simulink model "MPM"  (R2018b)
settings: Solver=VariableStepAuto  StartTime=0.0  StopTime=10.0  RelTol=1e-3
undefined symbols (not defined in the file): Cw, Cwc, Jt, Jw, k1, k2, k3, k4, Mt, R3, R4, Rg, Rw
settings Model: Creator=HYJ  LastModifiedBy=HYJ

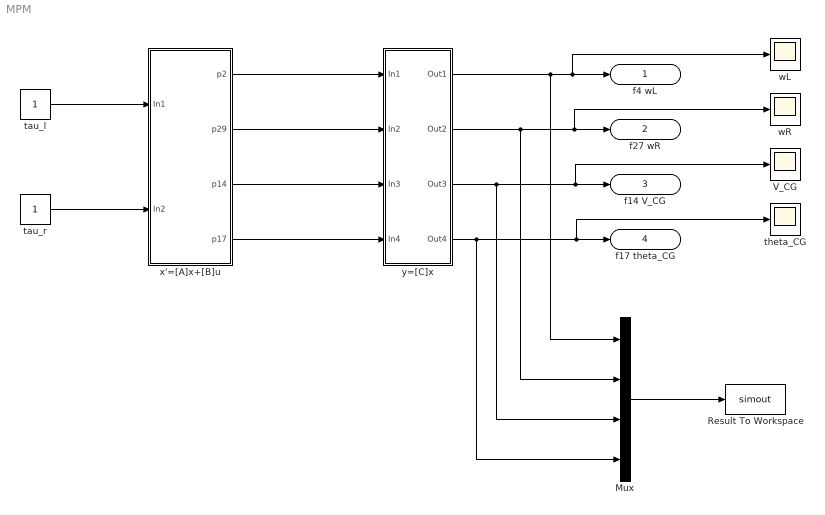
== system MPM ==
  Mux : Mux
  Result To Workspace : ToWorkspace  VariableName=simout  SaveFormat=Timeseries  SampleTime=-1
  V_CG : Scope
  tau_l : Constant
  tau_r : Constant
  theta_CG : Scope
  wL : Scope
  wR : Scope
  x'=[A]x+[B]u : Subsystem
  y=[C]x : Subsystem  mask{Jw=0, Mt=0, Jt=0}
  f4 wL : Outport
  f27 wR : Outport  Port=2
  f14 V_CG : Outport  Port=3
  f17 theta_CG : Outport  Port=4
  wires:
  tau_l/1 -> x'=[A]x+[B]u/1(In1)
  tau_r/1 -> x'=[A]x+[B]u/2(In2)
  y=[C]x/3(Out3) -> Mux/3, V_CG/1, f14 V_CG/1
  y=[C]x/2(Out2) -> Mux/2, wR/1, f27 wR/1
  y=[C]x/4(Out4) -> Mux/4, theta_CG/1, f17 theta_CG/1
  y=[C]x/1(Out1) -> Mux/1, wL/1, f4 wL/1
  x'=[A]x+[B]u/1(p2) -> y=[C]x/1(In1)
  x'=[A]x+[B]u/2(p29) -> y=[C]x/2(In2)
  x'=[A]x+[B]u/3(p14) -> y=[C]x/3(In3)
  x'=[A]x+[B]u/4(p17) -> y=[C]x/4(In4)
  Mux/1 -> Result To Workspace/1

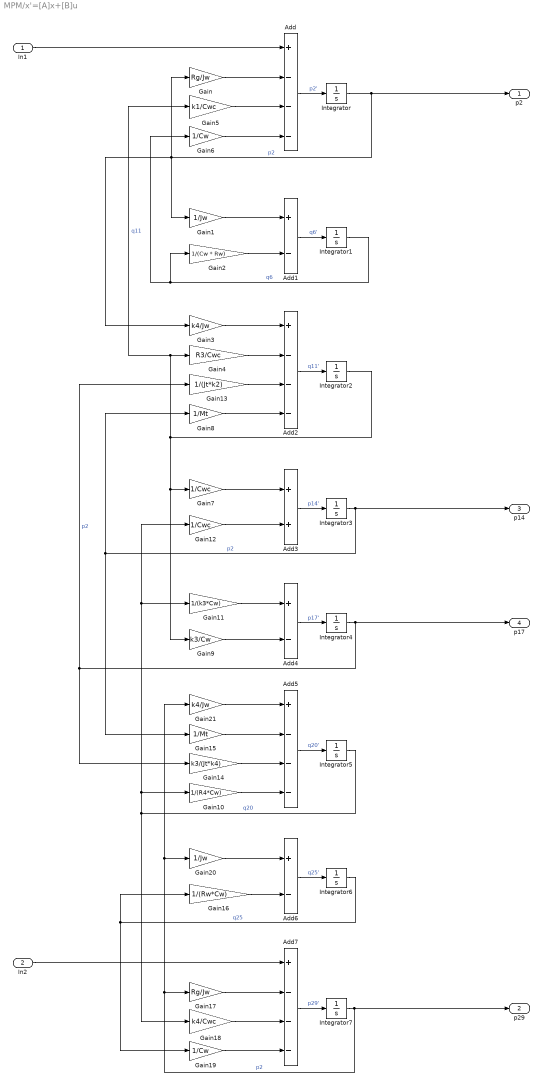
== system MPM/x'=[A]x+[B]u ==
  In1 : Inport
  In2 : Inport  Port=2
  Add{,2,5,7} (4 alike) : Sum  Inputs=+---
  Add1 : Sum  Inputs=+-
  Add3 : Sum
  Add4 : Sum  Inputs=+-
  Add6 : Sum  Inputs=+-
  Gain : Gain  Gain=Rg/Jw
  Gain1 : Gain  Gain=1/Jw
  Gain10 : Gain  Gain=1/(R4*Cw)
  Gain11 : Gain  Gain=1/(k3*Cw)
  Gain12 : Gain  Gain=1/Cwc
  Gain13 : Gain  Gain=1/(Jt*k2)
  Gain14 : Gain  Gain=k3/(Jt*k4)
  Gain15 : Gain  Gain=1/Mt
  Gain16 : Gain  Gain=1/(Rw*Cw)
  Gain17 : Gain  Gain=Rg/Jw
  Gain18 : Gain  Gain=k4/Cwc
  Gain19 : Gain  Gain=1/Cw
  Gain2 : Gain  Gain=1/(Cw * Rw)
  Gain20 : Gain  Gain=1/Jw
  Gain21 : Gain  Gain=k4/Jw
  Gain3 : Gain  Gain=k4/Jw
  Gain4 : Gain  Gain=R3/Cwc
  Gain5 : Gain  Gain=k1/Cwc
  Gain6 : Gain  Gain=1/Cw
  Gain7 : Gain  Gain=1/Cwc
  Gain8 : Gain  Gain=1/Mt
  Gain9 : Gain  Gain=k3/Cw
  Integrator{,1..7} (8 alike) : Integrator
  p2 : Outport
  p29 : Outport  Port=2
  p14 : Outport  Port=3
  p17 : Outport  Port=4
  wires:
  Add3/1 -> Integrator3/1  "p14'"
  Gain/1 -> Add/2
  In2/1 -> Add7/1
  Add7/1 -> Integrator7/1  "p29'"
  Integrator/1 -> p2/1, Gain3/1, Gain1/1, Gain/1  "p2"
  Integrator2/1 -> Gain9/1, Gain7/1, Gain5/1, Gain4/1  "q11"
  Add2/1 -> Integrator2/1  "q11'"
  Gain19/1 -> Add7/4
  Gain1/1 -> Add1/1
  Gain10/1 -> Add5/4
  Integrator1/1 -> Gain6/1, Gain2/1  "q6"
  Gain17/1 -> Add7/2
  Integrator5/1 -> Gain10/1, Gain12/1, Gain11/1, Gain18/1  "q20"
  Gain5/1 -> Add/3
  Add1/1 -> Integrator1/1  "q6'"
  Gain20/1 -> Add6/1
  Gain6/1 -> Add/4
  Gain11/1 -> Add4/1
  Add4/1 -> Integrator4/1  "p17'"
  Gain16/1 -> Add6/2
  Gain18/1 -> Add7/3
  Gain14/1 -> Add5/3
  Add/1 -> Integrator/1  "p2'"
  Gain2/1 -> Add1/2
  Gain9/1 -> Add4/2
  Gain15/1 -> Add5/2
  Gain8/1 -> Add2/4
  Integrator6/1 -> Gain19/1, Gain16/1  "q25"
  Gain3/1 -> Add2/1
  Gain13/1 -> Add2/3
  Gain4/1 -> Add2/2
  Add5/1 -> Integrator5/1  "q20'"
  Gain21/1 -> Add5/1
  Gain7/1 -> Add3/1
  Gain12/1 -> Add3/2
  In1/1 -> Add/1
  Add6/1 -> Integrator6/1  "q25'"
  Integrator3/1 -> p14/1, Gain8/1, Gain15/1  "p2"
  Integrator7/1 -> p29/1, Gain21/1, Gain20/1, Gain17/1  "p2"
  Integrator4/1 -> p17/1, Gain13/1, Gain14/1  "p2"

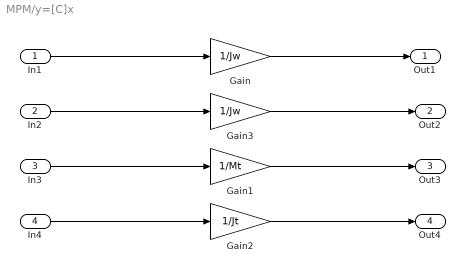
== system MPM/y=[C]x ==
  In1 : Inport
  In2 : Inport  Port=2
  In3 : Inport  Port=3
  In4 : Inport  Port=4
  Gain : Gain  Gain=1/Jw
  Gain1 : Gain  Gain=1/Mt
  Gain2 : Gain  Gain=1/Jt
  Gain3 : Gain  Gain=1/Jw
  Out1 : Outport
  Out2 : Outport  Port=2
  Out3 : Outport  Port=3
  Out4 : Outport  Port=4
  wires:
  Gain3/1 -> Out2/1
  In3/1 -> Gain1/1
  Gain2/1 -> Out4/1
  Gain/1 -> Out1/1
  Gain1/1 -> Out3/1
  In4/1 -> Gain2/1
  In2/1 -> Gain3/1
  In1/1 -> Gain/1
